simulink model "Unilat_Cntrl_LeadRob_Testing_Force"  (R2023b)
settings: Solver=FixedStepDiscrete  StartTime=0.0  StopTime=inf  FixedStep=0.002  RelTol=1e-3  EnableMultiTasking=on
libraries: quarc_library x2, simulink_extras x1
settings Model: SimulationMode=external  ExtModeTrigDuration=10000  Creator=Rchan  LastModifiedBy=angel
settings SolverCC: AlgebraicLoopSolver=TrustRegion  PositivePriorityOrder=on
settings DataIOCC: ReturnWorkspaceOutputs=off
settings DebuggingCC: UnconnectedInputMsg=warning  UnconnectedOutputMsg=warning  UnconnectedLineMsg=warning  ArithmeticOperatorsInVariantConditions=warning
settings ModelReferenceCC: EnableRefExpFcnMdlSchedulingChecks=on
settings SFSimCC: SimUseLocalCustomCode=off  CustomCodeUndefinedFunction=UseInterfaceOnly
settings RTWCC: Description=QUARC Win64 Target Using Toolchain  SystemTargetFile=quarc_win64.tlc  TemplateMakefile=quarc_default_tmf  RTWUseLocalCustomCode=off  Toolchain=QUARC win64 | nmake (64-bit Windows)  BuildConfiguration=Faster Runs
settings CodeAppCC: StateflowObjectComments=on
settings STFCustomTargetCC: ConcurrentExecutionCompliant=on  GRTInterface=on  UseToolchainInfoCompliant=on  SystemTargetFile=quarc_win64.tlc
settings GRTTargetCC: ParMdlRefBuildCompliant=off  CompOptLevelCompliant=off  CombineOutputUpdateFcns=off  MatFileLogging=off  CPPClassGenCompliant=off  GRTInterface=on  ExtMode=on  ExtModeMexFile=quarc_comm
settings ConfigComp: CovMetricSettings=dswe

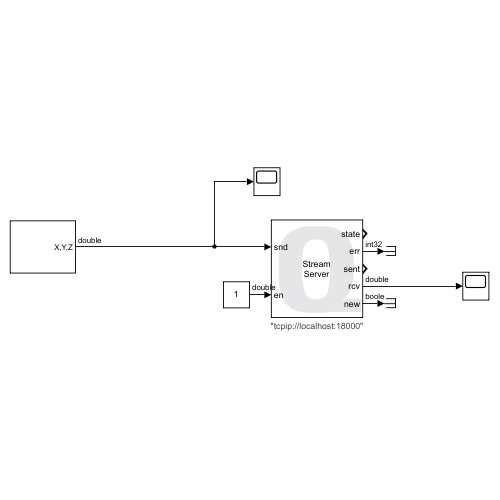
[thumbnail: Simulink's stored preview of the top-level diagram]
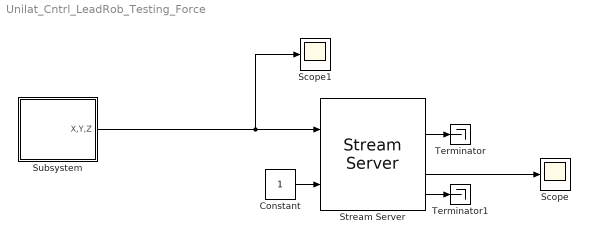
== system Unilat_Cntrl_LeadRob_Testing_Force ==
  Constant : Constant
  Scope : Scope
  Scope1 : Scope
  Stream Server : quarc_library/Communications/Basic/Stream Server  uri_source=Specify via dialog (do not evaluate)  uri=tcpip://localhost:18000  send_buffer_size=1460  receive_buffer_size=1460  byte_order=little endian (Intel - LSB first)  optimization=Minimum latency  send_options=Send all data  receive_options=Receive all data  default_value=[0 0]  sample_time=qc_get_step_size  active=on  implementation=Use blocking I/O in a separate thread  send_fifo_size=1000  receive_fifo_size=1000  send_priority=0  receive_priority=0  send_dimensions=off  receive_dimensions=off  max_dimensions=-1  data_type=Inherited via back propagation  type_expr=BusObject
      settings: AttributesFormatString="\"tcpip://localhost:18000\""
  Subsystem : Subsystem
  Terminator : Terminator
  Terminator1 : Terminator
  wires:
  Constant/1 -> Stream Server/2
  Stream Server/2 -> Terminator/1
  Stream Server/5 -> Terminator1/1
  Stream Server/4 -> Scope/1
  Subsystem/1(X,Y,Z) -> Scope1/1, Stream Server/1

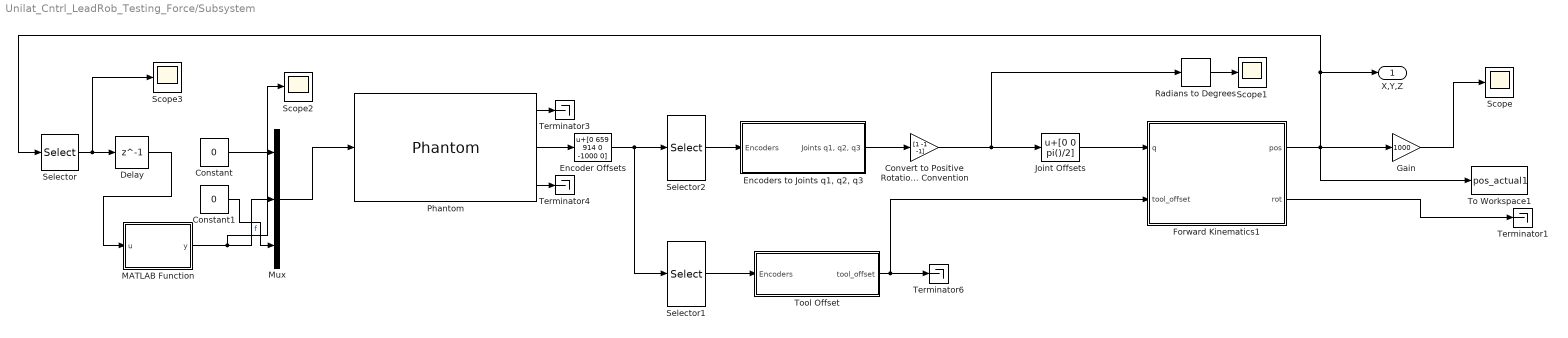
== system Unilat_Cntrl_LeadRob_Testing_Force/Subsystem ==
  Constant : Constant  Value=0
  Constant1 : Constant  Value=0
  Convert to Positive Rotation Convention : Gain  Gain=[1 -1 -1]
  Delay : Delay  DelayLength=1
  Encoder Offsets : Bias  Bias=[0 659 914 0 -1000 0]  SaturateOnIntegerOverflow=off
  "Encoders to Joints q1, q2, q3" : Subsystem
  Forward Kinematics1 : MATLAB Function  TreatAsAtomicUnit=on
  Gain : Gain  Gain=1000
  Joint Offsets : Bias  Bias=[0 0 pi()/2]  SaturateOnIntegerOverflow=off
  MATLAB Function : MATLAB Function  TreatAsAtomicUnit=on
  Mux : Mux  Inputs=3
  Phantom : quarc_library/Devices/Third-Party/SensAble/Phantom/Phantom  device_name=Default Device  output_type=Encoders Values  input_type=Joint space  velocity_limit_option=on  velocity_limit=1200  is_7dof=off  sample_time=-1
      settings: AttributesFormatString=(%<device_name>)  SourceProductName=QUARC Targets
  Radians to Degrees : simulink_extras/Transformations/Radians to Degrees
  Scope{,1..3} (4 alike) : Scope
  Selector : Selector  InputPortWidth=3  IndexOptions=Index vector (dialog)  Indices=[1]  OutputSizes=1
  Selector1 : Selector  InputPortWidth=6  IndexOptions=Index vector (dialog)  Indices=[4:6]  OutputSizes=1
  Selector2 : Selector  InputPortWidth=6  IndexOptions=Index vector (dialog)  Indices=[1:3]  OutputSizes=1
  Terminator{1,3..4,6} (4 alike) : Terminator
  To Workspace1 : ToWorkspace  VariableName=pos_actual1  SampleTime=-1
  Tool Offset : MATLAB Function  TreatAsAtomicUnit=on
  X,Y,Z : Outport
  wires:
  Phantom/2 -> Encoder Offsets/1
  Encoder Offsets/1 -> Selector2/1, Selector1/1
  Selector2/1 -> "Encoders to Joints q1, q2, q3"/1(Encoders)
  Phantom/1 -> Terminator3/1
  Selector1/1 -> Tool Offset/1(Encoders)
  Mux/1 -> Phantom/1
  Phantom/3 -> Terminator4/1
  Forward Kinematics1/2(rot) -> Terminator1/1
  Tool Offset/1(tool_offset) -> Forward Kinematics1/2(tool_offset), Terminator6/1
  Forward Kinematics1/1(pos) -> Selector/1, X,Y,Z/1, Gain/1, To Workspace1/1
  Gain/1 -> Scope/1
  Convert to Positive Rotation Convention/1 -> Radians to Degrees/1, Joint Offsets/1
  "Encoders to Joints q1, q2, q3"/1("Joints q1, q2, q3") -> Convert to Positive Rotation Convention/1
  Joint Offsets/1 -> Forward Kinematics1/1(q)
  Radians to Degrees/1 -> Scope1/1
  Selector/1 -> Scope3/1, Delay/1
  Delay/1 -> MATLAB Function/1(u)
  Constant/1 -> Mux/1
  MATLAB Function/1(y) -> Scope2/1, Mux/2
  Constant1/1 -> Mux/3  "f"

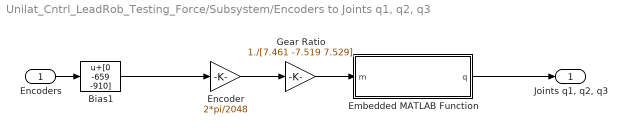
== system Unilat_Cntrl_LeadRob_Testing_Force/Subsystem/Encoders to Joints q1, q2, q3 ==
  Encoders : Inport
  Bias1 : Bias  Bias=[0 -659 -910]  SaturateOnIntegerOverflow=off
  Embedded MATLAB Function : MATLAB Function  TreatAsAtomicUnit=on
  Encoder : Gain  Gain=2*pi/2048
  Gear Ratio : Gain  Gain=1./[7.461 -7.519 7.529]
  "Joints q1, q2, q3" : Outport
  wires:
  Embedded MATLAB Function/1(q) -> "Joints q1, q2, q3"/1
  Encoders/1 -> Bias1/1
  Encoder/1 -> Gear Ratio/1
  Gear Ratio/1 -> Embedded MATLAB Function/1(m)
  Bias1/1 -> Encoder/1

== matlab function Unilat_Cntrl_LeadRob_Testing_Force/Subsystem/Tool Offset ==
  data: Encoders input; tool_offset output
function tool_offset = getToolOffset(Encoders)

%convert encoder values to angles using bias and gain
bias = [-2048 -2654 -2048];
gain = [2*pi()/4915 2*pi()/4096 2*pi()/4915];
Angle = (Encoders' + bias).*gain;

% convert the angle to the positive rotation convention defined
% by DH parameters
pos_rot = [-1 1 1];
joint_offset = [0 -(40-180)*pi/180 0];
Joint456 = Angle.*pos_rot + joint_offset;

%pick off theta4 and theta5
theta4 = Joint456(1);
theta5 = Joint456(2);

% The orientation of the tool offset matrix is given two successive
% rotations about x and z axis. 
RotZ = [cos(theta5) -sin(theta5) 0; sin(theta5) cos(theta5) 0; 0 0 1];
RotX = [1 0 0; 0 cos(theta4) -sin(theta4); 0 sin(theta4) cos(theta4)];
R = RotX*RotZ; % R is the rotation matrix of the tool offset matrix with respect to frame 3

% with respect to frame 3, the tool is 0.039m in the x-direction. Convert
% this vector to tool frame coordinates
tool_pos =R * [.039; 0; 0];

%create a Tool_offset transformation matrix. Use Identity matrix for
%rotation to show that the end effector frame and frame 3 are always
%aligned
I = [1 0 0; 0 1 0; 0 0 1];
tool = cat(2,I,tool_pos);
tool_offset = cat(1,tool,[0 0 0 1]);

== matlab function Unilat_Cntrl_LeadRob_Testing_Force/Subsystem/MATLAB Function ==
  data: u input; y output
function y = fcn(u)
if u > .15
    y = -0.25;
else
    y = 0;
end

== matlab function Unilat_Cntrl_LeadRob_Testing_Force/Subsystem/Encoders to Joints q1, q2, q3/Embedded MATLAB Function ==
  data: m input; q output
function q = Motors_2_Joints(m)
q = m;
q(1) = m(1);
q(2) = m(2);
q(3) = m(3) - m(2) -pi/2;
end

== matlab function Unilat_Cntrl_LeadRob_Testing_Force/Subsystem/Forward Kinematics1 ==
  data: pos output; q input; rot output; tool_offset input
function [pos,rot]    = ForwardKinematics(q,tool_offset)
% This block supports the Embedded MATLAB subset.
% See the help menu for details. 

% Link lengths
L1 = .132;
L2 = .132;

%Define A-matrices
%A1= DH(theta ,d ,a ,alpha)
A1 = DH(q(1), 0, 0, -pi()/2);
A2 = DH(q(2), 0, L1, 0);
A3 = DH(q(3)-pi/2, 0, L2, 0);

%Define T Matrices
T01=A1;
T02=T01*A2;
T03=T02*A3;

%tool_offset given with respect to frame 3.
T_tool=T03*tool_offset;
rot=T_tool(1:3,1:3);
pos=T_tool(1:3,4);


end

function A = DH(theta, d, a, alpha)

A_R_z = [cos(theta) -sin(theta) 0 0;
         sin(theta) cos(theta) 0 0;
         0 0 1 0;
         0 0 0 1];

A_T_z = [1 0 0 0;
         0 1 0 0;
         0 0 1 d;
         0 0 0 1];
     
  

A_T_x = [1 0 0 a;
         0 1 0 0;
         0 0 1 0;
         0 0 0 1];

A_R_x = [1 0 0 0;
         0 cos(alpha) -sin(alpha)  0;
         0 sin(alpha) cos(alpha) 0;
         0 0 0 1];

A = A_R_z*A_T_z*A_T_x*A_R_x;

end
